simulink model "TH31"  (R2018b)
settings: Solver=VariableStepAuto  StartTime=0.0  StopTime=10  RelTol=1e-3
settings Model: Creator=ohara  LastModifiedBy=ohara

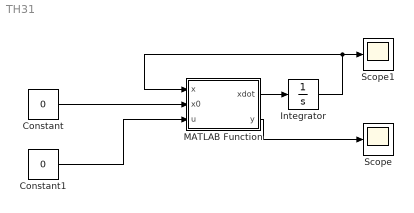
== system TH31 ==
  Constant : Constant  Value=0
  Constant1 : Constant  Value=0
  Integrator : Integrator  InitialCondition=[3,3,0]
  MATLAB Function : MATLAB Function  TreatAsAtomicUnit=on
  Scope : Scope
  Scope1 : Scope
  wires:
  Integrator/1 -> MATLAB Function/1(x), Scope1/1
  MATLAB Function/1(xdot) -> Integrator/1
  MATLAB Function/2(y) -> Scope/1
  Constant/1 -> MATLAB Function/2(x0)
  Constant1/1 -> MATLAB Function/3(u)

== matlab function TH31/MATLAB Function ==
  data: x input; x0 input; xdot output; u input; y output
function [xdot, y] = TH3(x, x0, u)
xdot1 = -3*x(1) +   x(2) + u;
xdot2 =    x(1) - 2*x(2) - x(3);
xdot3 =    x(2) - 3*x(3) + x0;
xdot  =   [xdot1 ; xdot2 ; xdot3];
y     =    x(3);
